simulink model "SimulinkDroneWorld"  (R2020a)
settings: Solver=VariableStepAuto  StartTime=0.0  StopTime=77  RelTol=1e-3
libraries: vrlib x1
settings Model: Creator=rjvar  LastModifiedBy=rjvar

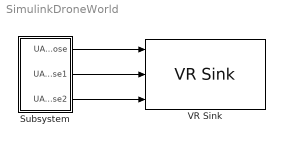
== system SimulinkDroneWorld ==
  Subsystem : Subsystem
  VR Sink : vrlib/VR Sink  InstantiateOnLoad=on  SampleTime=0.05  ViewEnable=on  RemoteChange=off  RemoteView=off  FieldsWritten=Drone1.translation.3.1.1.double#Drone2.translation.3.1.1.double#Drone3.translation.3.1.1.double  WorldFileName=C:\Users\rjvar\Dropbox\My PC (LAPTOP-HLU14FS6)\Desktop\Disaster_Prob.x3d  AutoView=off  VideoDimensions=[]  AllowVariableSize=off
  wires:
  Subsystem/1(UAV Pose) -> VR Sink/1
  Subsystem/2(UAV Pose1) -> VR Sink/2
  Subsystem/3(UAV Pose2) -> VR Sink/3

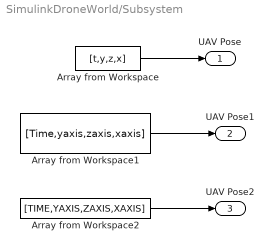
== system SimulinkDroneWorld/Subsystem ==
  Array from Workspace : FromWorkspace  VariableName=[t,y,z,x]
  Array from Workspace1 : FromWorkspace  VariableName=[Time,yaxis,zaxis,xaxis]
  Array from Workspace2 : FromWorkspace  VariableName=[TIME,YAXIS,ZAXIS,XAXIS]
  UAV Pose : Outport  VectorParamsAs1DForOutWhenUnconnected=off
  UAV Pose1 : Outport  Port=2  VectorParamsAs1DForOutWhenUnconnected=off
  UAV Pose2 : Outport  Port=3  VectorParamsAs1DForOutWhenUnconnected=off
  wires:
  Array from Workspace/1 -> UAV Pose/1
  Array from Workspace1/1 -> UAV Pose1/1
  Array from Workspace2/1 -> UAV Pose2/1
